simulink model "BESS_PassiveModel"  (R2018b)
settings: Solver=VariableStepAuto  StartTime=0.0  StopTime=1400  MaxStep=0.01  MinStep=0.00005  RelTol=1e-3
undefined symbols (not defined in the file or in its folder): Ion, Lithium
libraries: powerlib x4, electricdrivelib x1
settings Model: Creator=ttran  LastModifiedBy=ttran
settings SolverCC: ZeroCrossControl=EnableAll
settings DebuggingCC: IgnoredZcDiagnostic=none  SolverPrmCheckMsg=warning

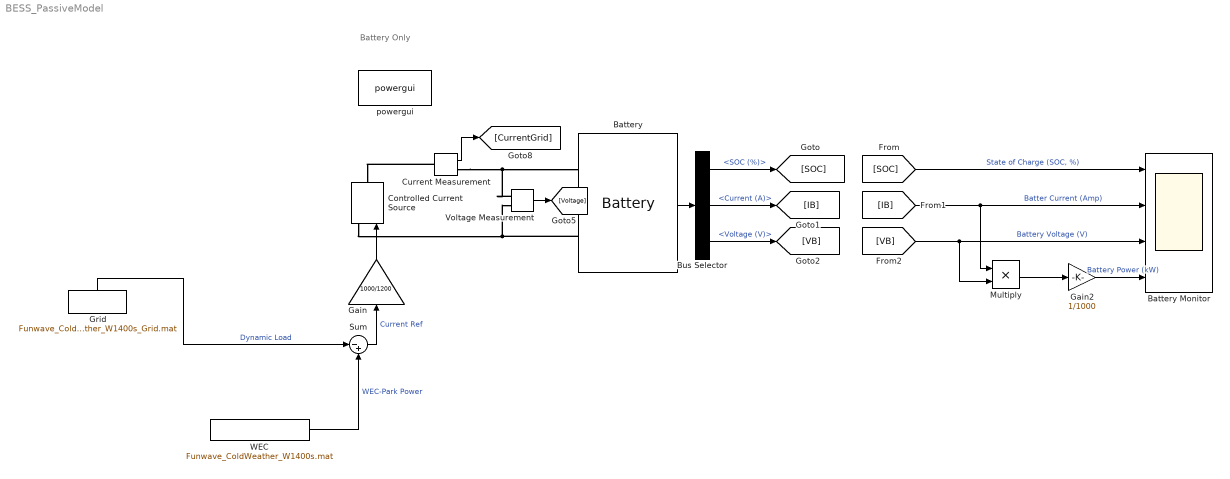
== system BESS_PassiveModel ==
  note: Battery Only
  Battery : electricdrivelib/Extra Sources/Battery  BatType=Lithium-Ion  ShowTempParam=off  ThermalPreset=no  ShowAgeParam=off  NomV=340  NomQ=100  SOC=50  Batt_Tr=1e-4  PresetModel=on  MaxQ=100  MinV=255  FullV=395.7556  Dis_rate=43.4783  R=0.034  Normal_OP=90.4348  expZone="[367.3312      4.913043]"  current=[6.5 13 32.5]  Units=Time  Tci=20  NomT=20  T2=-30  MaxQ2=4.8  FullV2=7.1  Normal_OP2=5.655  expZone2="[6.58           1]"  Rca=0.6  ti=2000  Dp=0  Neq0=0  Tsim=1e6  Ta1=25  Qeol=5.4*0.9  Reol=0.013333*1.2  Char_age=[2.3478, 3]  Dis_age=[2.3478, 10]  N1=1500  N2=10500  N3=1000  N4=1400  Ta2=45  N5=950
  Battery Monitor : Scope  NumInputPorts=4
  Bus Selector : BusSelector  OutputSignals=SOC (%),Current (A),Voltage (V)
  Controlled Current Source : powerlib/Electrical Sources/Controlled Current Source  Initialize=on  Source_Type=AC  Amplitude=0  Phase=0  Frequency=0  Measurements=None
  Current Measurement : powerlib/Measurements/Current Measurement  PhasorSimulation=off  OutputType=Complex  PSBequivalent=0
  Gain : Gain  Gain=1000/1200
  Gain2 : Gain  Gain=1/1000
  Grid : FromFile  FileName=Funwave_ColdWeather_W1400s_Grid.mat  SampleTime=0
  Multiply : Product
  Sum : Sum  Inputs=|-+
  Voltage Measurement : powerlib/Measurements/Voltage Measurement  PhasorSimulation=off  OutputType=Complex  PSBequivalent=0
  WEC : FromFile  FileName=Funwave_ColdWeather_W1400s.mat  SampleTime=0
  powergui : powerlib/powergui  Priority=1  SimulationMode=Continuous  SampleTime=50e-6  frequency=60  Iterations=50  frequencyindice=0  Pbase=100e6  ErrMax=1e-4  UnitsV=kV  UnitsW=MW  buscounter=0  FunctionMessages=off  echomessages=off  EnableUseOfTLC=off  CurrentSourceSwitches=off  DisableSnubberDevices=off  DisableRonSwitches=off  DisableVfSwitches=off  DisplayEquations=off  SolverType=Tustin/Backward Euler (TBE)  Interpol=off  ExternalGateDelay=off  methode=off  Ts=100  x0status=blocks  SPID=on  SwTol=0  HookPort=off  RestoreLinks=warning  ResistiveCurrentMeasurement=off  Frange=[0:2:500]  Ylog=off  Xlog=on  ShowGrid=off  save=off  variable=ZData  structure=0  ZoomFFT=off  StartTime=0.0  cycles=1  DisplayStyle=1  fundamental=60  FreqAxis=off  MaxFrequency=1000  frequencyindicesteady=1  RmsSteady=1  display=off
  wires:
  Battery/1 -> Bus Selector/1
  Bus Selector/1 -> [SOC]  "<SOC (%)>"
  Bus Selector/2 -> [IB]  "<Current (A)>"
  Bus Selector/3 -> [VB]  "<Voltage (V)>"
  [SOC] -> Battery Monitor/1  "State of Charge (SOC, %)"
  [IB] -> Battery Monitor/2, Multiply/1  "Batter Current (Amp)"
  [VB] -> Multiply/2, Battery Monitor/3  "Battery Voltage (V)"
  Multiply/1 -> Gain2/1
  Voltage Measurement/1 -> [Voltage]
  Current Measurement/1 -> [CurrentGrid]
  Grid/1 -> Sum/1  "Dynamic Load"
  Gain2/1 -> Battery Monitor/4  "Battery Power (kW)"
  WEC/1 -> Sum/2  "WEC-Park Power"
  Gain/1 -> Controlled Current Source/1
  Sum/1 -> Gain/1  "Current Ref"
  connections:
  Battery/LConn2 -- Controlled Current Source/LConn1 -- Voltage Measurement/LConn2
  Current Measurement/LConn1 -- Controlled Current Source/RConn1
  Voltage Measurement/LConn1 -- Current Measurement/RConn1 -- Battery/LConn1
